simulink model "Regen4"  (Simulink 6.5)
settings: Solver=FixedStepDiscrete  StartTime=0.0  StopTime=2  FixedStep=Ts  RelTol=1e-3  AbsTol=1e-3
PreLoadFcn:
  | assignin('base','Ts',[2e-6])
undefined symbols (not defined in the file): DiscIntNeverNeededParam, powergui, Ts
libraries: powerlib x21, powerlib_extras x6, simulink x2
settings Model: Creator=sybille  LastModifiedBy=RS  ExtModeTrigMode=oneshot  ExtModeArmWhenConnect=off  ExtModeAutoUpdateStatusClock=off
settings DataIOCC: LimitDataPoints=off  SaveOutput=off  SaveTime=off  SignalLoggingName=sigsOut
settings OptimizationCC: BlockReduction=off  BooleanDataType=off  InlineInvariantSignals=on
settings DebuggingCC: CheckExecutionContextPreStartOutputMsg=on  CheckExecutionContextRuntimeOutputMsg=on  SolverPrmCheckMsg=none  MultiTaskDSMMsg=warning  MultiTaskCondExecSysMsg=none  StrictBusMsg=None
settings HardwareCC: TargetUnknown=on
settings RTWCC: IncludeERTFirstTime=on

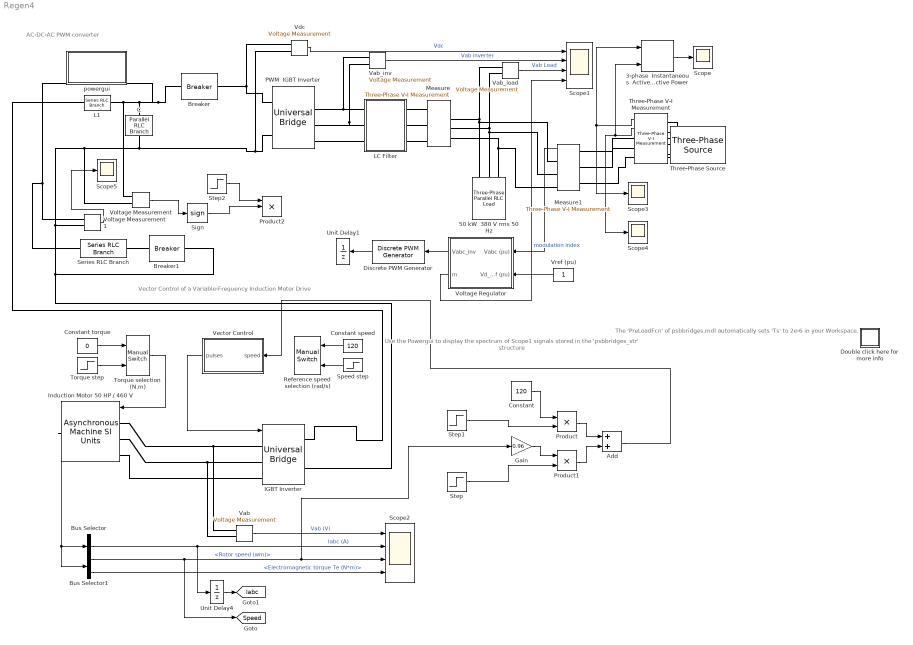
== system Regen4 ==
  note: AC-DC-AC PWM converter
  note: The 'PreLoadFcn' of psbbridges.mdl
      | automatically sets 'Ts' to 2e-6 in your Workspace.
  note: Use the Powergui to display
      | the spectrum of Scope1 signals
      | stored in the  'psbbridges_str'
      | structure
  note: Vector Control of a Variable-Frequency Induction Motor Drive
  3-phase  Instantaneous  Active & Reactive Power : powerlib_extras/Measurements/3-phase  Instantaneous  Active & Reactive Power  DialogController=PMDialogs.PMDefaultMaskDlg  SystemSampleTime=-1
  50 kW  380 V rms 50 Hz : powerlib/Elements/Three-Phase Parallel RLC Load  Orientation=down  DialogController=PMDialogs.PMDefaultMaskDlg  PhysicalDomain=powersysdomain  SubClassName=unknown  LeftPortType=p1  RightPortType=p1  LConnTagsString=A|B|C  Configuration=Y (grounded)  NominalVoltage=380  NominalFrequency=50  ActivePower=0  InductivePower=0  CapacitivePower=0  Measurements=None
  Add : Sum  OutScaling=2^-10
  Breaker : powerlib/Elements/Breaker  DialogController=PMDialogs.PMDefaultMaskDlg  SystemSampleTime=-1  BreakerResistance=0.01  InitialState=1  SnubberResistance=1e6  SnubberCapacitance=inf  SwitchingTimes=2  External=off  Measurements=None  MoreParameters=off  NoBreakLoop=off
  Breaker1 : powerlib/Elements/Breaker  DialogController=PMDialogs.PMDefaultMaskDlg  SystemSampleTime=-1  BreakerResistance=0.01  InitialState=0  SnubberResistance=1e6  SnubberCapacitance=inf  SwitchingTimes=2  External=off  Measurements=None  MoreParameters=off  NoBreakLoop=off
  Bus Selector : BusSelector  OutputSignals=Stator measurements.Stator current is_a (A),Stator measurements.Stator current is_b (A),Stator measurements.Stator current is_c (A)  OutputAsBus=on
  Bus Selector1 : BusSelector  OutputSignals=Mechanical.Rotor speed (wm),Mechanical.Electromagnetic torque Te (N*m)
  C : powerlib/Elements/Parallel RLC Branch  Orientation=down  DialogController=PMDialogs.PMDefaultMaskDlg  PhysicalDomain=powersysdomain  SubClassName=unknown  LeftPortType=p1  RightPortType=p1  LConnTagsString=a  RConnTagsString=__new0  BranchType=C  Resistance=1.0  Inductance=1.0  SetiL0=off  InitialCurrent=0  Capacitance=5000e-06  Setx0=off  InitialVoltage=0  Measurements=None
  Constant : Constant  Value=120  OutDataType=sfix(16)  ConRadixGroup=Use specified scaling  OutScaling=2^0  SampleTime=inf  FramePeriod=inf
  Constant speed : Constant  Orientation=left  Value=120  OutDataType=sfix(16)  ConRadixGroup=Use specified scaling  OutScaling=2^0  SampleTime=inf  FramePeriod=inf
  Constant torque : Constant  Value=0  OutDataType=sfix(16)  ConRadixGroup=Use specified scaling  OutScaling=2^0  SampleTime=inf  FramePeriod=inf
  Discrete PWM Generator : powerlib_extras/Discrete  Control Blocks/Discrete PWM Generator  Orientation=left  DialogController=PMDialogs.PMDefaultMaskDlg  SystemSampleTime=-1  GeneratorMode="3-arm  bridge (6 pulses)"  Fc=2000  Ts=Ts  Internal=off  mIndex=0.4  Freq=60  Phase=0
  Double click here for more info : Subsystem
      settings: OpenFcn=showdemo(bdroot(gcb))
      mask Display: disp('?')
  Gain : Gain  Gain=0.96
  IGBT Inverter : powerlib/Power Electronics/Universal Bridge  DialogController=PMDialogs.PMDefaultMaskDlg  SystemSampleTime=-1  Arms=3  SnubberResistance=1000  SnubberCapacitance=inf  Device=IGBT / Diodes  Ron=1e-3  Lon=0  ForwardVoltages="[  0.8  0.8  ]"  ForwardVoltage=.8  GTOparameters=[ 1e-6 , 1e-6 ]  IGBTparameters=[ 1e-6 , 2e-6 ]  Measurements=None  converterType=Rectifier
  Induction Motor 50 HP / 460 V : powerlib/Machines/Asynchronous Machine SI Units  Orientation=left  DialogController=PMDialogs.PMDefaultMaskDlg  SystemSampleTime=-1  PresetModel=No  MechanicalLoad=Torque Tm  ShowDetailedParameters=on  RotorType=Squirrel-cage  ReferenceFrame=Stationary  NominalParameters=[ 50*746, 460, 60 ]  Stator=[ 0.087 0.8e-3 ]  Rotor="[ 0.228  0.8e-3 ]"  Lm=34.7e-3  Mechanical="[0.2  0.04   2 ]"  PolePairs=2  InitialConditions="[ 1, 0 ,  0 , 0 , 0 , 0 , 0 , 0 ]"  Units=1  LoadFlowParameters=0  SimulateSaturation=off  Saturation=[0 0;0 0]
  L1 : powerlib/Elements/Series RLC Branch  DialogController=PMDialogs.PMDefaultMaskDlg  PhysicalDomain=powersysdomain  SubClassName=unknown  LeftPortType=p1  RightPortType=p1  LConnTagsString=__new0  RConnTagsString=__new0  BranchType=L  Resistance=1.0  Inductance=200e-6  SetiL0=off  InitialCurrent=0  Capacitance=1.0  Setx0=off  InitialVoltage=0  Measurements=None
  LC Filter : Subsystem
  Measure : powerlib/Measurements/Three-Phase V-I Measurement  DialogController=PMDialogs.PMDefaultMaskDlg  SystemSampleTime=-1  VoltageMeasurement=phase-to-ground  SetLabelV=off  LabelV=V1  Vpu=on  CurrentMeasurement=no  SetLabelI=off  LabelI=I1  Ipu=off  Pbase=1e3  Vbase=380  OutputType=Magnitude  PhasorSimulation=off  PSBequivalent=0
  Measure1 : powerlib/Measurements/Three-Phase V-I Measurement  Orientation=left  DialogController=PMDialogs.PMDefaultMaskDlg  SystemSampleTime=-1  VoltageMeasurement=phase-to-ground  SetLabelV=off  LabelV=V1  Vpu=on  CurrentMeasurement=no  SetLabelI=off  LabelI=I1  Ipu=off  Pbase=1e3  Vbase=500  OutputType=Magnitude  PhasorSimulation=off  PSBequivalent=0
  PWM  IGBT Inverter : powerlib/Power Electronics/Universal Bridge  Orientation=left  DialogController=PMDialogs.PMDefaultMaskDlg  SystemSampleTime=-1  Arms=3  SnubberResistance=5000  SnubberCapacitance=inf  Device=IGBT / Diodes  Ron=1e-3  Lon=0  ForwardVoltages="[  0.0  0.0  ]"  ForwardVoltage=.8  GTOparameters=[ 1e-6 ,1e-6 ]  IGBTparameters=[ 1e-6 , 2e-6 ]  Measurements=Device currents  converterType=Rectifier
  Product : Product  RndMeth=Zero
  Product1 : Product  RndMeth=Zero
  Product2 : Product  Inputs=3  RndMeth=Zero
  Reference speed selection (rad/s) : simulink/Signal Routing/Manual Switch  Orientation=left  SystemSampleTime=-1  sw=1  action=0
  Scope{,3..5} (4 alike) : Scope
      Scope settings: MaxDataPoints=10000000  SampleInput=on  SampleTime=2e-6
      Scope3 settings: SaveName=ScopeData2  MaxDataPoints=10000000  SampleInput=on  SampleTime=2e-6
      Scope4 settings: SaveName=ScopeData3  MaxDataPoints=10000000  SampleInput=on  SampleTime=2e-6
      Scope5 settings: SaveName=ScopeData4  MaxDataPoints=10000000  SampleInput=on  SampleTime=2e-6
  Scope1 : Scope  NumInputPorts=4
      settings: TimeRange=0.1  YMin=0~-1500~-750~0.4  YMax=1100~1500~750~1.1  SaveName=psbbridges_str
  Scope2 : Scope  NumInputPorts=4
      settings: TimeRange=3  YMin=-10000~-40~134~-70  YMax=10000~40~136.25~60  MaxDataPoints=100000000  Decimation=20  SampleInput=on  SampleTime=2e-6
  Series RLC Branch : powerlib/Elements/Series RLC Branch  DialogController=PMDialogs.PMDefaultMaskDlg  PhysicalDomain=powersysdomain  SubClassName=unknown  LeftPortType=p1  RightPortType=p1  LConnTagsString=__new0  RConnTagsString=__new0  BranchType=R  Resistance=40  Inductance=1e-3  SetiL0=off  InitialCurrent=0  Capacitance=1e-6  Setx0=off  InitialVoltage=0  Measurements=None
  Sign : Signum
  Speed step : Step  Orientation=left  Time=0.2  Before=120  After=160  SampleTime=0
  Step : Step  Time=0.7  SampleTime=0
  Step1 : Step  Time=0.7  Before=1  After=0  SampleTime=0
  Step2 : Step  Time=0.7  SampleTime=0
  Three-Phase V-I Measurement : powerlib/Measurements/Three-Phase V-I Measurement  Orientation=left  DialogController=PMDialogs.PMDefaultMaskDlg  SystemSampleTime=-1  VoltageMeasurement=phase-to-ground  SetLabelV=off  LabelV=Vabc  Vpu=off  CurrentMeasurement=yes  SetLabelI=off  LabelI=Iabc  Ipu=off  Pbase=100e6  Vbase=500e3  OutputType=Complex  PhasorSimulation=off  PSBequivalent=0
  Three-Phase Source : powerlib/Electrical Sources/Three-Phase Source  Orientation=left  DialogController=PMDialogs.PMDefaultMaskDlg  SystemSampleTime=-1  Voltage=500  PhaseAngle=5  Frequency=50  InternalConnection=Yg  SpecifyImpedance=off  Resistance=0.01  Inductance=0.001  ShortCircuitLevel=100e6  BaseVoltage=25e3  XRratio=7
  Torque selection (N.m) : simulink/Signal Routing/Manual Switch  SystemSampleTime=-1  sw=1  action=0
  Torque step : Step  Time=1.8  After=200  SampleTime=0
  Unit Delay1 : UnitDelay  Orientation=left  SampleTime=Ts
  Unit Delay4 : UnitDelay  SampleTime=Ts
  Vab : powerlib/Measurements/Voltage Measurement  Tag=PoWeRsYsTeMmEaSuReMeNt  DialogController=PMDialogs.PMDefaultMaskDlg  SystemSampleTime=-1  PhasorSimulation=off  OutputType=Magnitude  PSBequivalent=0
  Vab_inv : powerlib/Measurements/Voltage Measurement  Tag=PoWeRsYsTeMmEaSuReMeNt  DialogController=PMDialogs.PMDefaultMaskDlg  SystemSampleTime=-1  PhasorSimulation=off  OutputType=Magnitude  PSBequivalent=0
  Vab_load : powerlib/Measurements/Voltage Measurement  Tag=PoWeRsYsTeMmEaSuReMeNt  DialogController=PMDialogs.PMDefaultMaskDlg  SystemSampleTime=-1  PhasorSimulation=off  OutputType=Magnitude  PSBequivalent=0
  Vdc : powerlib/Measurements/Voltage Measurement  Tag=PoWeRsYsTeMmEaSuReMeNt  DialogController=PMDialogs.PMDefaultMaskDlg  SystemSampleTime=-1  PhasorSimulation=off  OutputType=Magnitude  PSBequivalent=0
  Vector Control : Subsystem  Orientation=left
  Voltage Measurement : powerlib/Measurements/Voltage Measurement  DialogController=PMDialogs.PMDefaultMaskDlg  SystemSampleTime=-1  PhasorSimulation=off  OutputType=Complex  PSBequivalent=0
  Voltage Measurement1 : powerlib/Measurements/Voltage Measurement  DialogController=PMDialogs.PMDefaultMaskDlg  SystemSampleTime=-1  PhasorSimulation=off  OutputType=Complex  PSBequivalent=0
  Voltage Regulator : Subsystem  Orientation=left  mask( Voltage Regulator){Kp=0.4, Ki=500, Ts=Ts}
      mask prompts: Kp "Proportional gain  Kp:"; Ki "Integral gain Ki:"; Ts "Sample time (s) :"
  "Vref (pu) " : Constant  Orientation=left  Value=1  OutDataType=sfix(16)  ConRadixGroup=Use specified scaling  OutScaling=2^0  SampleTime=inf  FramePeriod=inf
  powergui : Subsystem  Priority=2  AncestorBlock=powerlib/powergui  InitFcn=powergui( 'InitFcn_Callback' , gcb , 0 , [ ] );  mask(PSB option menu block){SimulationMode=Discrete, SampleTime=Ts, echomessages=off, RestoreLinks=warning, x0status=blocks, Frange=[0:2:500], Ylog=off, Xlog=on, ShowGrid=off, save=off, variable=ZData, structure=, ZoomFFT=on, StartTime=0.0, cycles=1, DisplayStyle=off, fundamental=60, FreqAxis=off, MaxFrequency=1000, frequencyindice=60, frequencyindicesteady=1, RmsSteady=1, display=off, Ts=0, frequency=60, methode=off, HookPort=off, Interpol=off}
      mask prompts: SimulationMode "Simulation mode"; SampleTime "Sample time Ts (when simulation mode is Discrete) (s)"; echomessages "Echo  Messages"; RestoreLinks "Restore disabled links"; x0status "Initial electrical states status"; Frange "Impedance tool: Frequency Range"; Ylog "Impedance tool: Log impedance"; Xlog "Impedance tool: log Frequency"; ShowGrid "Impedance tool: grid"; save "Impedance tool: Save Data To Workspace"; variable "Impedance tool: Variable Name"; structure "Structure Name (PSBFFTSCOPE)"; ZoomFFT "ZoomFFT (PSBFFTSCOPE)"; StartTime "Start Time (PSBFFTSCOPE)"; cycles "Cycles (PSBFFTSCOPE)"; DisplayStyle "Display style (PSBFFTSCOPE)"; fundamental "Fundamental (PSBFFTSCOPE)"; FreqAxis "Frequency Axis (PSBFFTSCOPE)"; MaxFrequency "Max Frequency (PSBFFTSCOPE)"; frequencyindice "Load flow frequency (Hz)"; frequencyindicesteady "Frequency indice (STEADYSTATE)"; RmsSteady "RMS display (STEADYSTATE)"; display "Display Results"; Ts "OBSOLETE 1"; frequency "Phasor frequency (Hz)"; methode "Phasor simulation"; HookPort "Hook port"; Interpol "Interpolate"
      mask init:
      | powerlibroot = which('powersysdomain');
      | PSBroot = powerlibroot(1:end-16);
      | %
      | switch SimulationMode
      | 	case 1
      | 		message=sprintf('Continuous');
      | 	case 2
      |         SampleTimeeval=evalin('base',SampleTime,'NaN');
      |         if isnan(SampleTimeeval)
      |             message=sprintf('Warning !!,\nUndefined sample time');
      |         else
      |             message=sprintf('Discrete,\nTs = %.4g s.',SampleTimeeval);
      |         end
      | 	case 3
      | 		message=sprintf('Phasors');
      | end
      | if strcmp(bdroot,'powerlib')
      |   message='powergui';
      | end
      | power_initmask();
      settings: CopyFcn=powergui( 'Copy_Callback' , gcb , 0 , [ ] );  ModelCloseFcn=powergui( 'CloseButton_Callback' , gcb , [ ] , [ ] );  PreSaveFcn=powergui( 'CloseButton_Callback' , gcb , [ ] , [ ] );  NameChangeFcn=powergui( 'NameChangeFcn_Callback' , gcb , 0 , [ ] );
      settings: DeleteFcn=|
      | powergui( 'Copy_Callback' , gcb , 1 , [ ] );
      | powergui( 'CloseButton_Callback' , gcb , [ ] , [ ] );
      settings: OpenFcn=|
      | if (power_openblockproxy ('secondary'))
      | powergui(gcb,'PM')
      | end;
      mask Help: web(psbhelp)
      mask StyleString: popup(Continuous|Discrete|Phasor),edit,checkbox,popup(yes|warning|no),popup(blocks|steady|zero),edit,checkbox,checkbox,checkbox,checkbox,edit,edit,checkbox,edit,edit,edit,edit,checkbox,edit,edit,edit,edit,checkbox,edit,edit,checkbox,checkbox,checkbox
      mask CallbackString: ||||||||||||||||||||||||||powergui('HookPort',[],[],gcb);|
      mask Display: disp(message)
  tag scope: Iabc=global, Speed=global
  wires:
  "Vref (pu) "/1 -> Voltage Regulator/2(Vd_ref (pu))
  Discrete PWM Generator/1 -> Unit Delay1/1
  Voltage Regulator/1(Vabc_inv) -> Discrete PWM Generator/1
  Voltage Regulator/2(m) -> Scope1/4  "modulation index"
  Vdc/1 -> Scope1/1  "Vdc"
  Vab_load/1 -> Scope1/3  "Vab Load"
  Vab_inv/1 -> Scope1/2  "Vab inverter"
  3-phase  Instantaneous  Active & Reactive Power/1 -> Scope/1
  Three-Phase V-I Measurement/1 -> Scope3/1, 3-phase  Instantaneous  Active & Reactive Power/1
  Three-Phase V-I Measurement/2 -> Scope4/1, 3-phase  Instantaneous  Active & Reactive Power/2
  Measure1/1 -> Voltage Regulator/1(Vabc (pu))
  Bus Selector1/1 -> [Speed], Scope2/3, Gain/1  "<Rotor speed (wm)>"
  Vector Control/1(pulses) -> IGBT Inverter/1
  Torque step/1 -> Torque selection (N.m)/2
  Constant torque/1 -> Torque selection (N.m)/1
  Constant speed/1 -> Reference speed selection (rad/s)/1
  Speed step/1 -> Reference speed selection (rad/s)/2
  Bus Selector/1 -> Scope2/2, Unit Delay4/1  "Iabc (A)"
  Vab/1 -> Scope2/1  "Vab (V)"
  Bus Selector1/2 -> Scope2/4  "<Electromagnetic torque Te (N*m)>"
  Torque selection (N.m)/1 -> Induction Motor 50 HP / 460 V/1
  Induction Motor 50 HP / 460 V/1 -> Bus Selector1/1, Bus Selector/1
  Unit Delay4/1 -> [Iabc]
  Product1/1 -> Add/2
  Product/1 -> Add/1
  Constant/1 -> Product/1
  Gain/1 -> Product1/1
  Add/1 -> Vector Control/1(speed)
  Step1/1 -> Product/2
  Step/1 -> Product1/2
  Step2/1 -> Product2/1
  Voltage Measurement/1 -> Sign/1
  Sign/1 -> Product2/2
  Voltage Measurement1/1 -> Scope5/1
  connections:
  PWM  IGBT Inverter/RConn2 -- Vdc/LConn2 -- C/RConn1 -- Voltage Measurement/LConn2 -- IGBT Inverter/RConn2 -- Breaker1/RConn1 -- Voltage Measurement1/LConn2
  PWM  IGBT Inverter/RConn1 -- Vdc/LConn1 -- Breaker/RConn1
  Vab_inv/LConn2 -- PWM  IGBT Inverter/LConn2 -- LC Filter/LConn2
  Measure/RConn2 -- Vab_load/LConn2 -- 50 kW  380 V rms 50 Hz/LConn2 -- Measure1/RConn2
  Measure/RConn1 -- Vab_load/LConn1 -- 50 kW  380 V rms 50 Hz/LConn1 -- Measure1/RConn1
  50 kW  380 V rms 50 Hz/LConn3 -- Measure/RConn3 -- Measure1/RConn3
  Three-Phase Source/RConn1 -- Three-Phase V-I Measurement/LConn1
  Three-Phase Source/RConn2 -- Three-Phase V-I Measurement/LConn2
  Three-Phase Source/RConn3 -- Three-Phase V-I Measurement/LConn3
  PWM  IGBT Inverter/LConn1 -- Vab_inv/LConn1 -- LC Filter/LConn1
  LC Filter/LConn3 -- PWM  IGBT Inverter/LConn3
  LC Filter/RConn1 -- Measure/LConn1
  LC Filter/RConn2 -- Measure/LConn2
  LC Filter/RConn3 -- Measure/LConn3
  Measure1/LConn1 -- Three-Phase V-I Measurement/RConn1
  Measure1/LConn2 -- Three-Phase V-I Measurement/RConn2
  Three-Phase V-I Measurement/RConn3 -- Measure1/LConn3
  Vab/LConn2 -- Induction Motor 50 HP / 460 V/LConn2 -- IGBT Inverter/LConn2
  Vab/LConn1 -- Induction Motor 50 HP / 460 V/LConn1 -- IGBT Inverter/LConn1
  L1/LConn1 -- IGBT Inverter/RConn1
  IGBT Inverter/LConn3 -- Induction Motor 50 HP / 460 V/LConn3
  L1/RConn1 -- Voltage Measurement/LConn1 -- C/LConn1 -- Breaker/LConn1 -- Voltage Measurement1/LConn1 -- Series RLC Branch/LConn1
  Series RLC Branch/RConn1 -- Breaker1/LConn1

== system Regen4/Double click here for more info ==
  note: This example of AC-DC-AC converter illustrates use of Universal Bridge,
      | Multimeter, and Powergui  blocks, as well as discrete control blocks of the Extras library
  note: Circuit Description
  note: Demonstration
  note: A  60 Hz, voltage source feeds a 50 Hz, 50 kW load through an  AC-DC-AC  converter.
      |
      | The 600V, 60 Hz voltage obtained at secondary of the Wye/Delta transformer is first rectified by a six pulse diode bridge.
      | The filtered DC voltage is applied to an IGBT two-level inverter generating 50 Hz.
      | The IGBT inverter uses Pulse Width Modulation (PWM) at a 2 kHz carrier frequency.
      | The circuit is discretized at a sample time of 2 us
      |
      | The load voltage is regulated at 1 pu (380 V rms) by a PI voltage regulator using abc_to_dq and dq_to_abc transfomations.
      | The first output of the voltage regulator is a vector containing the three modulating signals used by the PMW Generator
      | to generate the 6 IGBT pulses. The second output returns the modulation index.
      |
      | The Discrete 3-Phase PWM Pulse Generator is available in the Extras/Discrete Control Blocks library.
      | The voltage regulator has been  built from blocks of the Extras/Measurements and Extras/ Discrete Control libraries
      |
      | The Multimeter block is used to observe diode and IGBT currents.
      | In order to allow further signal processing, signals displayed on  Scope1 block  (sampled at simulation sampling rate of 2us )
      | are stored in a  variable named 'psbbridges_str' (structure with time) .
  note: Start the simulation. After a transient period of approximately  50 ms, the system reaches a steady state.
      | Observe  voltage waveforms at  DC bus, inverter output  and load on Scope1.
      | The harmonics generated by the inverter around around multiples of 2 kHz are filtered by the  LC filter.
      |
      | As expected the peak value of the load voltage is 537 V (380 Vrms).
      | In steady state, the mean value of the modulation index is m = 0.80 and the mean value of the  DC  voltage is 778 V.
      | The fundamental component of 50 Hz voltage burried in the chopped inverter voltage is therefore:
      | Vab = 778 V * 0.612 * 0.80 = 381 V rms
      |
      | Once  simulation is completed, open the Powergui and select  'FFT Analysis' to display the 0 - 7000 Hz frequency spectrum of signals saved
      | in the 'psbbridges_str' structure. The FFT will be performed on  a 2-cycle window starting at t=0.1-2/50 (last 2 cycles of recording).
      | Select input labeled 'Vab Load' . Click on Display and observe the frequency spectrum of last 2 cycles.
      | Notice harmonics around multiples of the 2 kHz carrier frequency. Maximum harmonic is 1.4 % of fundamental and THD is 2%.
      |
      | Observe diode currents on trace 1 of Scope2, showing commutation from  diode 1 to diode 3.  Also observe on trace 2 currents in
      | switches 1 and 2 of the IGBT/Diode bridge (upper and lower switches connected to phase A). These two currents are complementary.
      | A positive current indicates a current flowing in the IGBT, whereas a negative current indicates a current flowing in the antiparallel diode.
  note: G. Sybille (Hydro-Quebec)

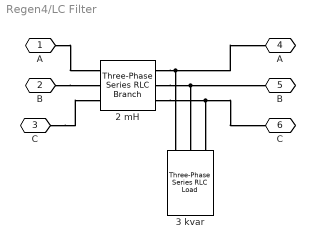
== system Regen4/LC Filter ==
  "2 mH " : powerlib/Elements/Three-Phase Series RLC Branch  DialogController=PMDialogs.PMDefaultMaskDlg  PhysicalDomain=powersysdomain  SubClassName=unknown  LeftPortType=p1  RightPortType=p1  LConnTagsString=A|B|C  RConnTagsString=A|B|C  BranchType=L  Resistance=1.0  Inductance=2e-3  Capacitance=1.0  Measurements=None
  3 kvar : powerlib/Elements/Three-Phase Series RLC Load  Orientation=down  DialogController=PMDialogs.PMDefaultMaskDlg  PhysicalDomain=powersysdomain  SubClassName=unknown  LeftPortType=p1  RightPortType=p1  LConnTagsString=A|B|C  Configuration=Y (grounded)  NominalVoltage=380  NominalFrequency=50  ActivePower=0  InductivePower=0  CapacitivePower=3e3  Measurements=None
  A : PMIOPort  Port=1  Side=Left
  B : PMIOPort  Port=2  Side=Left
  C : PMIOPort  Port=3  Side=Left
  "A " : PMIOPort  Orientation=left  Port=4  Side=Right
  "B " : PMIOPort  Orientation=left  Port=5  Side=Right
  "C " : PMIOPort  Orientation=left  Port=6  Side=Right
  connections:
  B/RConn1 -- "2 mH "/LConn2
  A/RConn1 -- "2 mH "/LConn1
  C/RConn1 -- "2 mH "/LConn3
  "2 mH "/RConn1 -- "A "/RConn1 -- 3 kvar/LConn1
  "2 mH "/RConn2 -- "B "/RConn1 -- 3 kvar/LConn2
  "2 mH "/RConn3 -- "C "/RConn1 -- 3 kvar/LConn3

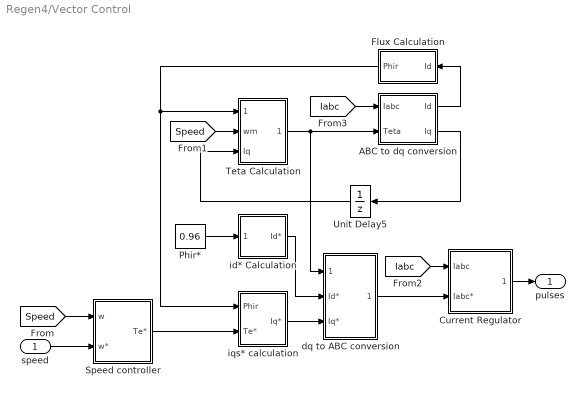
== system Regen4/Vector Control ==
  speed : Inport
  ABC to dq conversion : Subsystem
  Current Regulator : Subsystem  mask(Regulateur de courant a hysteresis){h=20}
      mask prompts: h "Hysteresis band (A)"
  Flux Calculation : Subsystem  Orientation=left  mask(Flux Calcultation){}
      mask init:
      | NF=0.44572610323020e-6;
      | DF=[1 -0.99998715486734];
  Phir* : Constant  Value=0.96  OutDataType=sfix(16)  ConRadixGroup=Use specified scaling  OutScaling=2^0  SampleTime=inf  FramePeriod=inf
  Speed controller : Subsystem  mask(PI controller){Kp=13, Ki=26, Tlim=300, Ts=Ts}
      mask prompts: Kp "Proportional gain (Kp)"; Ki "Integral gain (Ki)"; Tlim "Torque limit (N.m)"; Ts "Sampling time (s)"
      mask help: Proportional-Integral Speed Controller
      mask Display: plot(0,0,100,100,[35,35,65],[70,30,30],[35,65],[45,60])
  Teta Calculation : Subsystem
  Unit Delay5 : UnitDelay  Orientation=left  SampleTime=Ts
  dq to ABC conversion : Subsystem
  id* Calculation : Subsystem
  iqs* calculation : Subsystem
  pulses : Outport
  wires:
  dq to ABC conversion/1(Iabc*) -> Current Regulator/2(Iabc*)
  Speed controller/1(Te*) -> iqs* calculation/2(Te*)
  Phir*/1 -> id* Calculation/1(Phir*)
  ABC to dq conversion/1(Id) -> Flux Calculation/1(Id)
  id* Calculation/1(Id*) -> dq to ABC conversion/2(Id*)
  Flux Calculation/1(Phir) -> Teta Calculation/1(Phir), iqs* calculation/1(Phir)
  ABC to dq conversion/2(Iq) -> Unit Delay5/1
  Unit Delay5/1 -> Teta Calculation/3(Iq)
  iqs* calculation/1(Iq*) -> dq to ABC conversion/3(Iq*)
  Teta Calculation/1(Teta) -> dq to ABC conversion/1(Teta), ABC to dq conversion/2(Teta)
  [Speed] -> Speed controller/1(w)
  [Speed] -> Teta Calculation/2(wm)
  [Iabc] -> Current Regulator/1(Iabc)
  [Iabc] -> ABC to dq conversion/1(Iabc)
  speed/1 -> Speed controller/2(w*)
  Current Regulator/1(Pulses) -> pulses/1

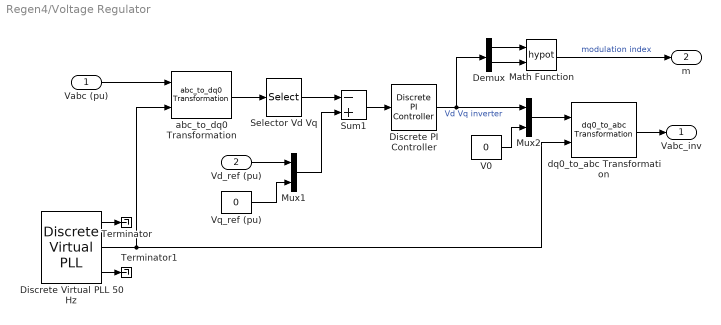
== system Regen4/Voltage Regulator ==
  Vabc (pu) : Inport
  Vd_ref (pu) : Inport  Port=2
  Demux : Demux  Outputs=2
  Discrete PI Controller : powerlib_extras/Discrete  Control Blocks/Discrete PI Controller  DialogController=PMDialogs.PMDefaultMaskDlg  SystemSampleTime=-1  Kp=Kp  Ki=Ki  Par_Limits=[1 -1]  Init=0  Ts=Ts
  Discrete Virtual PLL 50 Hz : powerlib_extras/Discrete  Control Blocks/Discrete Virtual PLL  DialogController=PMDialogs.PMDefaultMaskDlg  SystemSampleTime=-1  Freq=50  Phase=0  Ts=Ts
  Math Function : Math  Operator=hypot  SaturateOnIntegerOverflow=on
  Mux1 : Mux  Inputs=2
  Mux2 : Mux  Inputs=2
  Selector Vd Vq : Selector  InputType=Vector  ElementSrc=Internal  Elements=[1 2]  RowSrc=Internal  Rows=1  ColumnSrc=Internal  Columns=1  InputPortWidth=3  IndexIsStartValue=off
  Sum1 : Sum  Inputs=-+  SaturateOnIntegerOverflow=on  InputSameDT=on
  Terminator : Terminator
  Terminator1 : Terminator
  V0 : Constant  Value=0  OutDataType=sfix(16)  ConRadixGroup=Use specified scaling  OutScaling=2^0  SampleTime=inf  FramePeriod=inf
  Vq_ref (pu) : Constant  Value=0  OutDataType=sfix(16)  ConRadixGroup=Use specified scaling  OutScaling=2^0  SampleTime=inf  FramePeriod=inf
  abc_to_dq0 Transformation : powerlib_extras/Measurements/abc_to_dq0 Transformation  DialogController=PMDialogs.PMDefaultMaskDlg  SystemSampleTime=-1
  dq0_to_abc Transformation : powerlib_extras/Measurements/dq0_to_abc Transformation  DialogController=PMDialogs.PMDefaultMaskDlg  SystemSampleTime=-1
  Vabc_inv : Outport
  m : Outport  Port=2
  wires:
  abc_to_dq0 Transformation/1 -> Selector Vd Vq/1
  Vabc (pu)/1 -> abc_to_dq0 Transformation/1
  Selector Vd Vq/1 -> Sum1/1
  Sum1/1 -> Discrete PI Controller/1
  Mux2/1 -> dq0_to_abc Transformation/1
  V0/1 -> Mux2/2
  dq0_to_abc Transformation/1 -> Vabc_inv/1
  Discrete Virtual PLL 50 Hz/2 -> abc_to_dq0 Transformation/2, dq0_to_abc Transformation/2
  Vd_ref (pu)/1 -> Mux1/1
  Vq_ref (pu)/1 -> Mux1/2
  Mux1/1 -> Sum1/2
  Discrete Virtual PLL 50 Hz/1 -> Terminator/1
  Discrete Virtual PLL 50 Hz/3 -> Terminator1/1
  Discrete PI Controller/1 -> Demux/1, Mux2/1  "Vd Vq inverter"
  Demux/1 -> Math Function/1
  Demux/2 -> Math Function/2
  Math Function/1 -> m/1  "modulation index"

== system Regen4/powergui ==
  note: Graphical user interface for the analysis of  SimPowerSystems circuits.
      | Place the Powergui block in the top-level of your model and double-click
      | on it to open the GUI.
  EquivalentModel1 : Subsystem
      mask init:
      | SPS = get_param(gcbh,'UserData');
      | if isempty(SPS)
      | 	Ts=1;
      |     A=0;
      |     B=0;
      |     C=0;
      |     D=0;
      |     x0=0;
      |     SwitchResistance=1;
      |     SwitchType=1;
      |     SwitchGateInitialValue=1;
      |     OutputsToResetToZero=1;
      | else
      | 	Ts=SPS.PowerguiInfo.Ts;
      | 	A=SPS.Adiscrete;
      |     B=SPS.Bdiscrete;
      |     C=SPS.Cdiscrete;
      |     D=SPS.Ddiscrete;
      |     x0=SPS.x0discrete;
      |     SwitchResistance=SPS.SwitchResistance;
      |     SwitchType=SPS.SwitchType;
      |     SwitchGateInitialValue=SPS.SwitchGateInitialValue;
      |     OutputsToResetToZero=SPS.YSwitchCurrent;
      | end
      mask Display:
      | color('orange')
      | disp('EQUIVALENT CIRCUIT')
  Ground : Ground
  Terminator : Terminator
  wires:
  Ground/1 -> Terminator/1

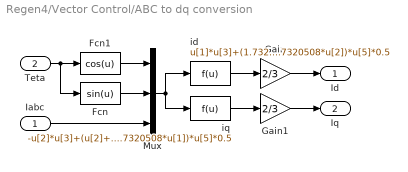
== system Regen4/Vector Control/ABC to dq conversion ==
  Iabc : Inport
  Teta : Inport  Port=2
  Fcn : Fcn  Expr=sin(u)
  Fcn1 : Fcn  Expr=cos(u)
  Gain : Gain  Gain=2/3  SaturateOnIntegerOverflow=on
  Gain1 : Gain  Gain=2/3  SaturateOnIntegerOverflow=on
  Mux : Mux  Inputs=[1 1 3]
  id : Fcn  Expr=u[1]*u[3]+(1.7320508*u[2]-u[1])*u[4]*0.5+(-u[1]-1.7320508*u[2])*u[5]*0.5
  iq : Fcn  Expr=-u[2]*u[3]+(u[2]+1.7320508*u[1])*u[4]*0.5+(u[2]-1.7320508*u[1])*u[5]*0.5
  Id : Outport  InitialOutput=0
  Iq : Outport  Port=2  InitialOutput=0
  wires:
  Fcn/1 -> Mux/2
  Fcn1/1 -> Mux/1
  Teta/1 -> Fcn1/1, Fcn/1
  Mux/1 -> iq/1, id/1
  Iabc/1 -> Mux/3
  iq/1 -> Gain1/1
  id/1 -> Gain/1
  Gain/1 -> Id/1
  Gain1/1 -> Iq/1

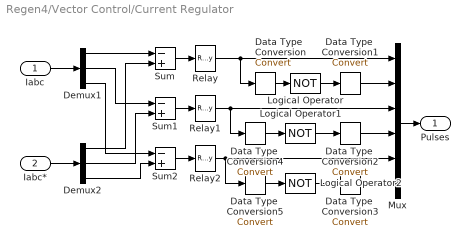
== system Regen4/Vector Control/Current Regulator ==
  Iabc : Inport
  Iabc* : Inport  Port=2
  Data Type  Conversion : DataTypeConversion  OutDataTypeMode=boolean  SaturateOnIntegerOverflow=on  RndMeth=Zero
  Data Type  Conversion1 : DataTypeConversion  OutDataTypeMode=double  SaturateOnIntegerOverflow=on  RndMeth=Zero
  Data Type  Conversion2 : DataTypeConversion  OutDataTypeMode=double  SaturateOnIntegerOverflow=on  RndMeth=Zero
  Data Type  Conversion3 : DataTypeConversion  OutDataTypeMode=double  SaturateOnIntegerOverflow=on  RndMeth=Zero
  Data Type  Conversion4 : DataTypeConversion  OutDataTypeMode=boolean  SaturateOnIntegerOverflow=on  RndMeth=Zero
  Data Type  Conversion5 : DataTypeConversion  OutDataTypeMode=boolean  SaturateOnIntegerOverflow=on  RndMeth=Zero
  Demux1 : Demux  Outputs=3
  Demux2 : Demux  Outputs=3
  Logical Operator : Logic  Operator=NOT
  Logical Operator1 : Logic  Operator=NOT
  Logical Operator2 : Logic  Operator=NOT
  Mux : Mux  Inputs=6
  Relay : Relay  OnSwitchValue=h/2  OffSwitchValue=-h/2
  Relay1 : Relay  OnSwitchValue=h/2  OffSwitchValue=-h/2
  Relay2 : Relay  OnSwitchValue=h/2  OffSwitchValue=-h/2
  Sum : Sum  Inputs=-+  SaturateOnIntegerOverflow=on  InputSameDT=on
  Sum1 : Sum  Inputs=-+  SaturateOnIntegerOverflow=on  InputSameDT=on
  Sum2 : Sum  Inputs=-+  SaturateOnIntegerOverflow=on  InputSameDT=on
  Pulses : Outport  InitialOutput=0
  wires:
  Sum/1 -> Relay/1
  Sum1/1 -> Relay1/1
  Demux1/1 -> Sum/1
  Demux1/2 -> Sum1/1
  Mux/1 -> Pulses/1
  Iabc/1 -> Demux1/1
  Sum2/1 -> Relay2/1
  Demux1/3 -> Sum2/1
  Demux2/3 -> Sum2/2
  Demux2/2 -> Sum1/2
  Demux2/1 -> Sum/2
  Iabc*/1 -> Demux2/1
  Relay/1 -> Mux/1, Data Type  Conversion/1
  Relay1/1 -> Mux/3, Data Type  Conversion4/1
  Relay2/1 -> Mux/5, Data Type  Conversion5/1
  Data Type  Conversion/1 -> Logical Operator/1
  Logical Operator/1 -> Data Type  Conversion1/1
  Data Type  Conversion1/1 -> Mux/2
  Logical Operator1/1 -> Data Type  Conversion2/1
  Data Type  Conversion2/1 -> Mux/4
  Logical Operator2/1 -> Data Type  Conversion3/1
  Data Type  Conversion3/1 -> Mux/6
  Data Type  Conversion4/1 -> Logical Operator1/1
  Data Type  Conversion5/1 -> Logical Operator2/1

== system Regen4/Vector Control/Flux Calculation ==
  note: Phir = Lm *Id / (1 +Tr .s)
  note: Lm = 34.7 mH
  note: Lr = Ll'r +Lm = 0.8 +34.7= 35.5 mH
  note: Tr = Lr / Rr = 0.1557 s
  note: Rr = 0.228 ohms
  Id : Inport  Orientation=left
  Discrete Tranfer Function : Subsystem  Orientation=left  mask(First Order Low Pass Filter (Discrete)){T=0.1557, Ts=Ts}
      mask prompts: T "Time constant T (s) :"; Ts "Time step (s)"
      mask help: H(s)=1/(1+T.s)
      mask init:
      | X=[0 1 2 3 4];
      |  Y=[-2 -2 -3 -4 -4];
      |  str=sprintf('\nH=1/(1+T.s)\n T= %g s\n\n\n',T);
      | num=1;
      | den=[T 1];
      | 
      | % discrete transfer function
      | % descending powers of z
      | numd= Ts/T;
      | dend=[ 1  (Ts-T)/T];
      mask Display:
      | plot(X,Y);
      | disp(str);
  Lm : Gain  Orientation=left  Gain=34.7e-3  SaturateOnIntegerOverflow=on
  Phir : Outport  Orientation=left
  wires:
  Discrete Tranfer Function/1(Out) -> Phir/1
  Id/1 -> Lm/1
  Lm/1 -> Discrete Tranfer Function/1(In)

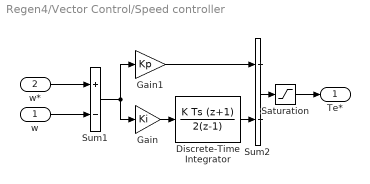
== system Regen4/Vector Control/Speed controller ==
  w : Inport
  w* : Inport  Port=2
  Discrete-Time Integrator : DiscreteIntegrator  IntegratorMethod=Integration: Trapezoidal  SampleTime=Ts  LimitOutput=on  UpperSaturationLimit=Tlim  LowerSaturationLimit=-Tlim  ICPrevOutput=DiscIntNeverNeededParam  ICPrevScaledInput=DiscIntNeverNeededParam
  Gain : Gain  Gain=Ki  SaturateOnIntegerOverflow=on
  Gain1 : Gain  Gain=Kp  SaturateOnIntegerOverflow=on
  Saturation : Saturate  UpperLimit=Tlim  LowerLimit=-Tlim
  Sum1 : Sum  Inputs=+-  SaturateOnIntegerOverflow=on  InputSameDT=on
  Sum2 : Sum  SaturateOnIntegerOverflow=on  InputSameDT=on
  Te* : Outport  InitialOutput=0
  wires:
  Gain1/1 -> Sum2/1
  Gain/1 -> Discrete-Time Integrator/1
  Sum1/1 -> Gain/1, Gain1/1
  Discrete-Time Integrator/1 -> Sum2/2
  Sum2/1 -> Saturation/1
  Saturation/1 -> Te*/1
  w/1 -> Sum1/2
  w*/1 -> Sum1/1

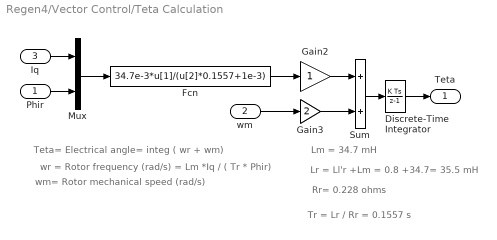
== system Regen4/Vector Control/Teta Calculation ==
  note: Teta= Electrical angle= integ ( wr + wm)
  note: wr = Rotor frequency (rad/s) = Lm *Iq / ( Tr * Phir)
  note: Lm = 34.7 mH
  note: Rr= 0.228 ohms
  note: Lr = Ll'r +Lm = 0.8 +34.7= 35.5 mH
  note: wm= Rotor mechanical speed (rad/s)
  note: Tr = Lr / Rr = 0.1557 s
  Phir : Inport
  wm : Inport  Port=2
  Iq : Inport  Port=3
  Discrete-Time Integrator : DiscreteIntegrator  SampleTime=Ts  ICPrevOutput=DiscIntNeverNeededParam  ICPrevScaledInput=DiscIntNeverNeededParam
  Fcn : Fcn  Expr=34.7e-3*u[1]/(u[2]*0.1557+1e-3)
  Gain2 : Gain  SaturateOnIntegerOverflow=on
  Gain3 : Gain  Gain=2  SaturateOnIntegerOverflow=on
  Mux : Mux  Inputs=2
  Sum : Sum  SaturateOnIntegerOverflow=on  InputSameDT=on
  Teta : Outport  InitialOutput=0
  wires:
  Discrete-Time Integrator/1 -> Teta/1
  Sum/1 -> Discrete-Time Integrator/1
  Gain3/1 -> Sum/2
  Gain2/1 -> Sum/1
  wm/1 -> Gain3/1
  Fcn/1 -> Gain2/1
  Phir/1 -> Mux/2
  Iq/1 -> Mux/1
  Mux/1 -> Fcn/1

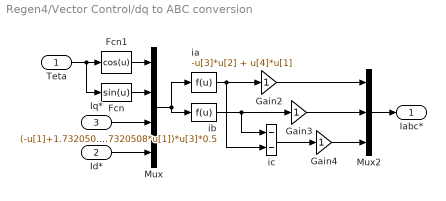
== system Regen4/Vector Control/dq to ABC conversion ==
  Teta : Inport
  Id* : Inport  Port=2
  Iq* : Inport  Port=3
  Fcn : Fcn  Expr=sin(u)
  Fcn1 : Fcn  Expr=cos(u)
  Gain2 : Gain  SaturateOnIntegerOverflow=on
  Gain3 : Gain  SaturateOnIntegerOverflow=on
  Gain4 : Gain  SaturateOnIntegerOverflow=on
  Mux : Mux
  Mux2 : Mux  Inputs=3
  ia : Fcn  Expr=-u[3]*u[2] + u[4]*u[1]
  ib : Fcn  Expr=(-u[1]+1.7320508*u[2])*u[4]*0.5+(u[2]+1.7320508*u[1])*u[3]*0.5
  ic : Sum  Inputs=--  SaturateOnIntegerOverflow=on  InputSameDT=on
  Iabc* : Outport  InitialOutput=0
  wires:
  Fcn/1 -> Mux/2
  Fcn1/1 -> Mux/1
  Mux2/1 -> Iabc*/1
  Mux/1 -> ib/1, ia/1
  Teta/1 -> Fcn1/1, Fcn/1
  Iq*/1 -> Mux/3
  Id*/1 -> Mux/4
  Gain3/1 -> Mux2/2
  ic/1 -> Gain4/1
  Gain4/1 -> Mux2/3
  Gain2/1 -> Mux2/1
  ia/1 -> Gain2/1, ic/2
  ib/1 -> Gain3/1, ic/1

== system Regen4/Vector Control/id* Calculation ==
  note: Id* = Phir*/ Lm
  note: Lm= 34.7 mH
  Phir* : Inport
  KF : Gain  Gain=1/34.7e-3  SaturateOnIntegerOverflow=on
  Id* : Outport
  wires:
  KF/1 -> Id*/1
  Phir*/1 -> KF/1

== system Regen4/Vector Control/iqs* calculation ==
  note: Iq= ( 2/3) * (2/p) * ( Lr/Lm) * (Te / Phir)
  note: Lm = 34.7 mH
  note: Lr = Ll'r +Lm = 0.8 +34.7= 35.5 mH
  note: p= nb of poles = 4
  note: Iq= 0.341 * (Te / Phir)
  Phir : Inport
  Te* : Inport  Port=2
  Fcn : Fcn  Expr=u[1]*0.341/(u[2]+1e-3)
  Mux1 : Mux  Inputs=2
  Iq* : Outport  InitialOutput=0
  wires:
  Phir/1 -> Mux1/2
  Fcn/1 -> Iq*/1
  Te*/1 -> Mux1/1
  Mux1/1 -> Fcn/1

== system Regen4/powergui/EquivalentModel1 ==
  Gates : Subsystem
  Sources : Subsystem
  State-Space : S-Function  FunctionName=sfun_spssw_discc  Parameters=Ts,A, B, C, D, x0, SwitchResistance ,SwitchType, SwitchGateInitialValue, OutputsToResetToZero
  Status : Subsystem
  Yout : Subsystem
  wires:
  State-Space/1 -> Yout/1(v,i)
  State-Space/2 -> Status/1(status)
  Sources/1(u) -> State-Space/1
  Gates/1(gates) -> State-Space/2

== system Regen4/Vector Control/Flux Calculation/Discrete Tranfer Function ==
  In : Inport
  Discrete Transfer Fcn : DiscreteTransferFcn  Numerator=numd  Denominator=dend  SampleTime=Ts
  Out : Outport  InitialOutput=0
  wires:
  Discrete Transfer Fcn/1 -> Out/1
  In/1 -> Discrete Transfer Fcn/1

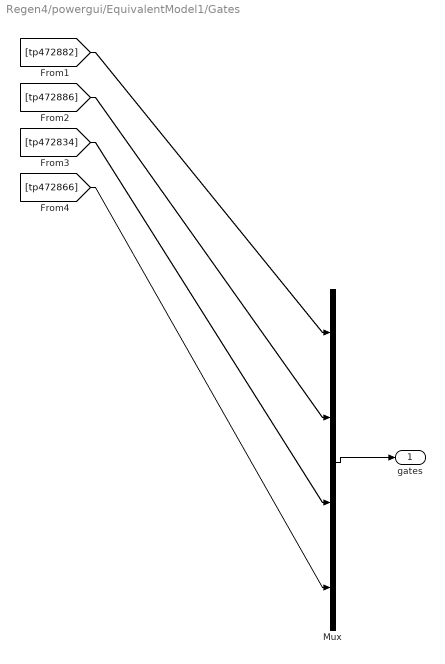
== system Regen4/powergui/EquivalentModel1/Gates ==
  Mux : Mux  Inputs=[1 1 6 6]
  gates : Outport
  wires:
  Mux/1 -> gates/1
  [tp472882] -> Mux/1
  [tp472886] -> Mux/2
  [tp472834] -> Mux/3
  [tp472866] -> Mux/4

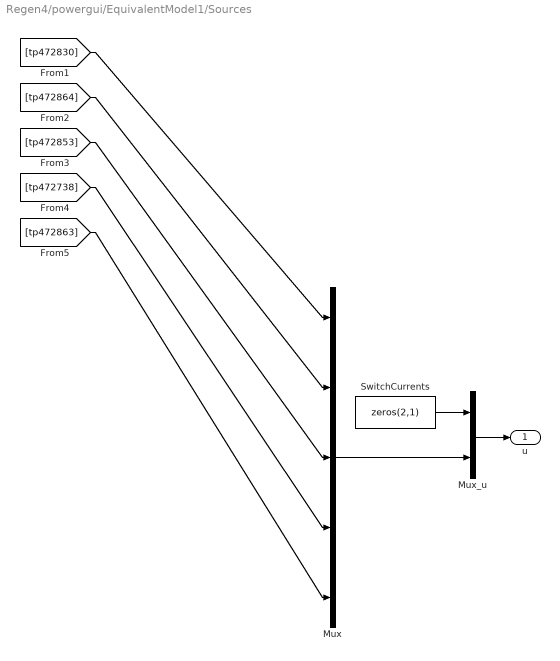
== system Regen4/powergui/EquivalentModel1/Sources ==
  Mux : Mux  Inputs=[6 6 2 3 6]
  Mux_u : Mux  Inputs=[2 23]
  SwitchCurrents : Constant  Value=zeros(2,1)  OutDataType=sfix(16)  ConRadixGroup=Use specified scaling  OutScaling=2^0  SampleTime=inf  FramePeriod=inf
  u : Outport
  wires:
  Mux/1 -> Mux_u/2
  SwitchCurrents/1 -> Mux_u/1
  Mux_u/1 -> u/1
  [tp472830] -> Mux/1
  [tp472864] -> Mux/2
  [tp472853] -> Mux/3
  [tp472738] -> Mux/4
  [tp472863] -> Mux/5

== system Regen4/powergui/EquivalentModel1/Status ==
  status : Inport
  Demux : Demux  Outputs=[1 1 6 6]
  tag scope: tp472835=global, tp472867=global, tp472883=global, tp472887=global
  wires:
  status/1 -> Demux/1
  Demux/1 -> [tp472883]
  Demux/2 -> [tp472887]
  Demux/3 -> [tp472835]
  Demux/4 -> [tp472867]

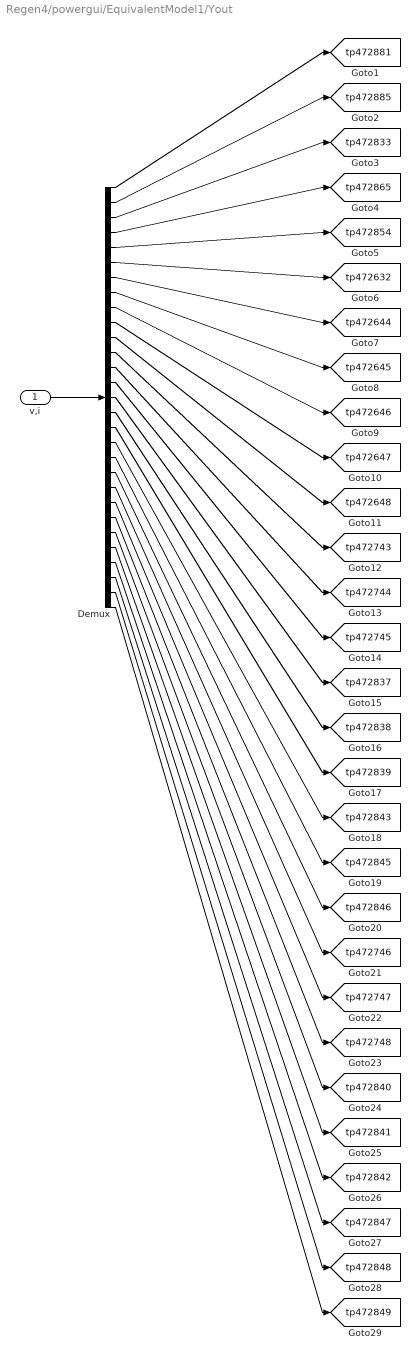
== system Regen4/powergui/EquivalentModel1/Yout ==
  v,i : Inport
  Demux : Demux  Outputs=[1 1 6 6 2 1 1 1 1 1 1 1 1 1 1 1 1 1 1 1 1 1 1 1 1 1 1 1 1]
  tag scope: tp472632=global, tp472644=global, tp472645=global, tp472646=global, tp472647=global, tp472648=global, tp472743=global, tp472744=global, tp472745=global, tp472746=global, tp472747=global, tp472748=global, tp472833=global, tp472837=global, tp472838=global, tp472839=global, tp472840=global, tp472841=global, tp472842=global, tp472843=global, tp472845=global, tp472846=global, tp472847=global, tp472848=global, tp472849=global, tp472854=global, tp472865=global, tp472881=global, tp472885=global
  wires:
  v,i/1 -> Demux/1
  Demux/1 -> [tp472881]
  Demux/2 -> [tp472885]
  Demux/3 -> [tp472833]
  Demux/4 -> [tp472865]
  Demux/5 -> [tp472854]
  Demux/6 -> [tp472632]
  Demux/7 -> [tp472644]
  Demux/8 -> [tp472645]
  Demux/9 -> [tp472646]
  Demux/10 -> [tp472647]
  Demux/11 -> [tp472648]
  Demux/12 -> [tp472743]
  Demux/13 -> [tp472744]
  Demux/14 -> [tp472745]
  Demux/15 -> [tp472837]
  Demux/16 -> [tp472838]
  Demux/17 -> [tp472839]
  Demux/18 -> [tp472843]
  Demux/19 -> [tp472845]
  Demux/20 -> [tp472846]
  Demux/21 -> [tp472746]
  Demux/22 -> [tp472747]
  Demux/23 -> [tp472748]
  Demux/24 -> [tp472840]
  Demux/25 -> [tp472841]
  Demux/26 -> [tp472842]
  Demux/27 -> [tp472847]
  Demux/28 -> [tp472848]
  Demux/29 -> [tp472849]
